simulink model "MainPendulum_Discrete"  (R2025b)
settings: Solver=VariableStepAuto  StartTime=0.0  StopTime=20.0  RelTol=1e-3
values from neighbouring files (symbols this model uses):
  Kx = dlqr(Ad, Bd, Qz_d, R_d)    [lqr_linear_discrete.m]
undefined symbols (not defined in the file or in its folder): Discrete, h, Time
libraries: simulink_extras x2, ctrlSharedLib x1
settings Model: Creator=djangovanderplas  LastModifiedBy=djangovanderplas

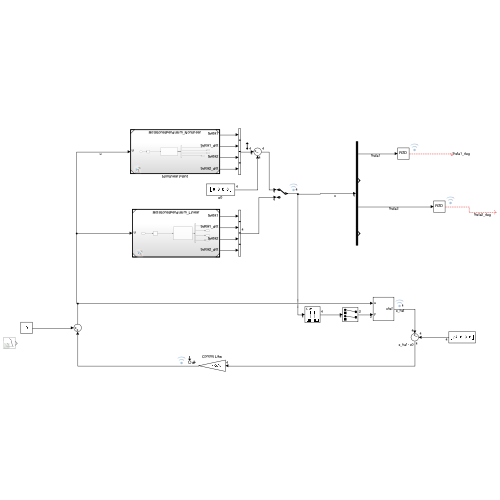
[thumbnail: Simulink's stored preview of the top-level diagram]
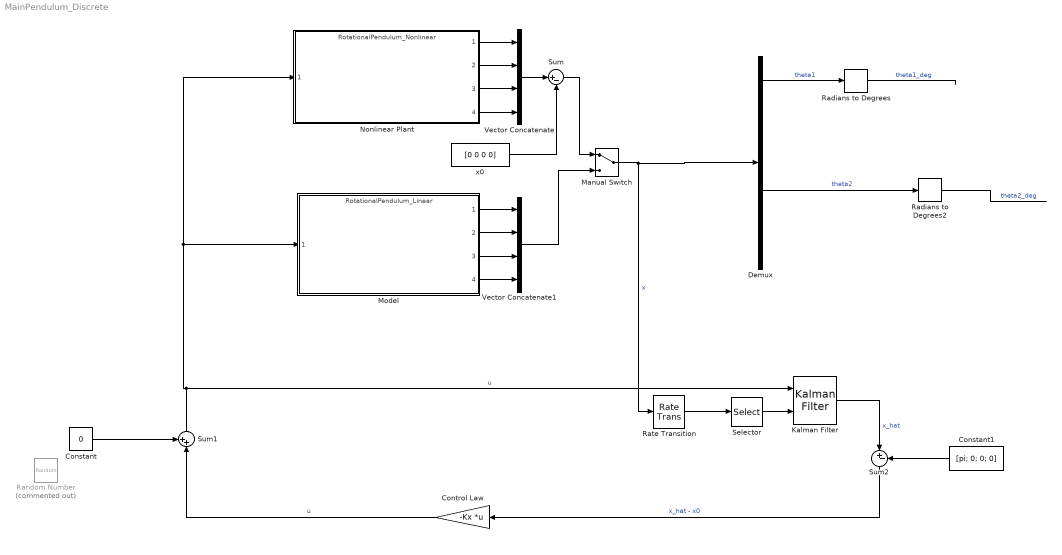
== system MainPendulum_Discrete ==
  Constant : Constant  Value=0  SampleTime=h
  Constant1 : Constant  Value=[pi; 0; 0; 0]  SampleTime=h
  Control Law : Gain  Gain=-Kx  Multiplication=Matrix(K*u)
  Demux : Demux
  Kalman Filter : ctrlSharedLib/Kalman Filter  TimeDomain=Discrete-Time  UseCurrentEstimator=on  ModelSource=LTI State-Space Variable  ModelSourceVariable=sys_kf_d  A=0.95  B=1  C=1  D=0  NumberOfStates=1  NumberOfInputs=1  NumberOfOutputs=1  InitialEstimateSource=Dialog  X0=[pi; 0; 0; 0];  P0=10  UseK=off  UseGH=off  NumberOfProcessNoiseInputs=1  G=1  TimeInvariantG=on  H=0  TimeInvariantH=on  Q=0.05*eye(4)  TimeInvariantQ=on  R=1*eye(2)  TimeInvariantR=on  N=zeros(4, 2)  TimeInvariantN=on  AddInputPort=on  AddEnablePort=off  OutputEstimatedY=off  OutputP=off  Ts=-1
  Manual Switch : ManualSwitch
  Model : ModelReference  ModelNameDialog=RotationalPendulum_Linear.slx  SimulationMode=Normal  ModelReferenceVersion=1.6
  Nonlinear Plant : ModelReference  ModelNameDialog=RotationalPendulum_Nonlinear  SimulationMode=Normal  ModelReferenceVersion=1.15
  Radians to Degrees : simulink_extras/Transformations/Radians to Degrees
  Radians to Degrees2 : simulink_extras/Transformations/Radians to Degrees
  Random Number : RandomNumber  Commented=on  Variance=0.01  SampleTime=0.1
  Rate Transition : RateTransition  OutPortSampleTime=h
  Selector : Selector  InputPortWidth=4  IndexOptions=Index vector (dialog)  Indices=[1 3]  OutputSizes=1
  Sum : Sum  Inputs=|+-
  Sum1 : Sum  Inputs=++|
  Sum2 : Sum  Inputs=|+-
  Vector Concatenate : Concatenate  NumInputs=4
  Vector Concatenate1 : Concatenate  NumInputs=4
  x0 : Constant  Value=[0 0 0 0]
  wires:
  Nonlinear Plant/1 -> Vector Concatenate/1
  Nonlinear Plant/2 -> Vector Concatenate/2
  Nonlinear Plant/3 -> Vector Concatenate/3
  Nonlinear Plant/4 -> Vector Concatenate/4
  Model/1 -> Vector Concatenate1/1
  Model/2 -> Vector Concatenate1/2
  Model/3 -> Vector Concatenate1/3
  Model/4 -> Vector Concatenate1/4
  Demux/1 -> Radians to Degrees/1  "theta1"
  Demux/3 -> Radians to Degrees2/1  "theta2"
  Vector Concatenate/1 -> Sum/1
  Sum/1 -> Manual Switch/1
  Manual Switch/1 -> Rate Transition/1, Demux/1  "x"
  Vector Concatenate1/1 -> Manual Switch/2
  x0/1 -> Sum/2
  Radians to Degrees/1 -> ?  "theta1_deg"
  Radians to Degrees2/1 -> ?  "theta2_deg"
  Sum1/1 -> Nonlinear Plant/1, Model/1, Kalman Filter/1  "u"
  Selector/1 -> Kalman Filter/2
  Control Law/1 -> Sum1/2  "u"
  Constant/1 -> Sum1/1
  Rate Transition/1 -> Selector/1
  Sum2/1 -> Control Law/1  "x_hat - x0"
  Kalman Filter/1 -> Sum2/1  "x_hat"
  Constant1/1 -> Sum2/2
